simulink subsystem "airframe_aerodynamics"  (R2023b)
settings: Solver=VariableStepAuto  StartTime=0.0  StopTime=10.0  RelTol=1e-3
undefined symbols (not defined in the file): b, c, C_D, C_l, C_L, C_m, C_n, C_Y, p, S
libraries: sharedtransform x1
settings Model: Creator=Victor  LastModifiedBy=Victor

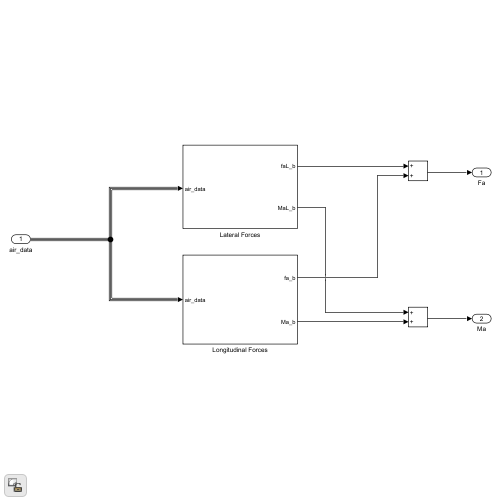
[thumbnail: Simulink's stored preview of the top-level diagram]
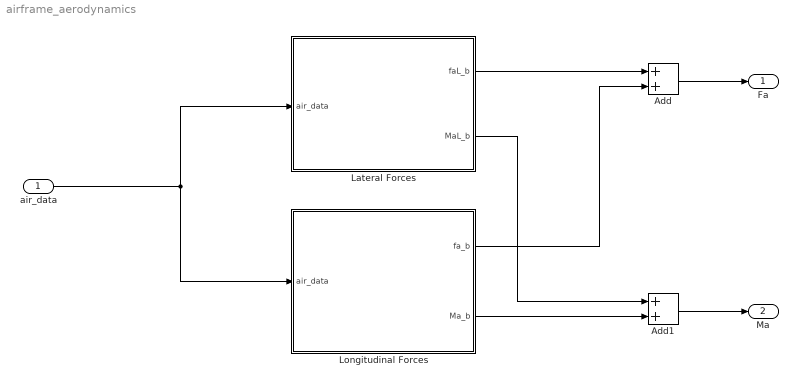
== system airframe_aerodynamics ==
  air_data : Inport
  Add : Sum
  Add1 : Sum
  Lateral Forces : Subsystem
  Longitudinal Forces : Subsystem
  Fa : Outport
  Ma : Outport  Port=2
  wires:
  air_data/1 -> Longitudinal Forces/1(air_data), Lateral Forces/1(air_data)
  Lateral Forces/1(faL_b) -> Add/1
  Longitudinal Forces/1(fa_b) -> Add/2
  Add/1 -> Fa/1
  Lateral Forces/2(MaL_b) -> Add1/1
  Longitudinal Forces/2(Ma_b) -> Add1/2
  Add1/1 -> Ma/1

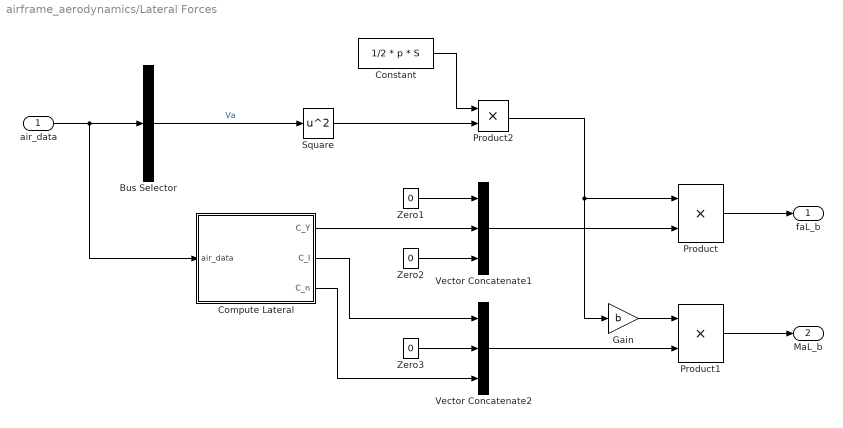
== system airframe_aerodynamics/Lateral Forces ==
  air_data : Inport
  Bus Selector : BusSelector  OutputSignals=target.Va  OutputAsBus=on
  Compute Lateral : Subsystem
  Constant : Constant  Value=1/2 * p * S
  Gain : Gain  Gain=b
  Product : Product
  Product1 : Product
  Product2 : Product
  Square : Math  Operator=square
  Vector Concatenate1 : Concatenate  NumInputs=3
  Vector Concatenate2 : Concatenate  NumInputs=3
  Zero1 : Constant  Value=0  OutDataTypeStr=Inherit: Inherit via back propagation
  Zero2 : Constant  Value=0  OutDataTypeStr=Inherit: Inherit via back propagation
  Zero3 : Constant  Value=0  OutDataTypeStr=Inherit: Inherit via back propagation
  faL_b : Outport
  MaL_b : Outport  Port=2
  wires:
  Bus Selector/1 -> Square/1  "Va"
  Product/1 -> faL_b/1
  air_data/1 -> Compute Lateral/1(air_data), Bus Selector/1
  Zero1/1 -> Vector Concatenate1/1
  Zero2/1 -> Vector Concatenate1/3
  Compute Lateral/1(C_Y) -> Vector Concatenate1/2
  Compute Lateral/3(C_n) -> Vector Concatenate2/3
  Compute Lateral/2(C_l) -> Vector Concatenate2/1
  Zero3/1 -> Vector Concatenate2/2
  Product1/1 -> MaL_b/1
  Square/1 -> Product2/2
  Constant/1 -> Product2/1
  Product2/1 -> Gain/1, Product/1
  Vector Concatenate1/1 -> Product/2
  Vector Concatenate2/1 -> Product1/2
  Gain/1 -> Product1/1

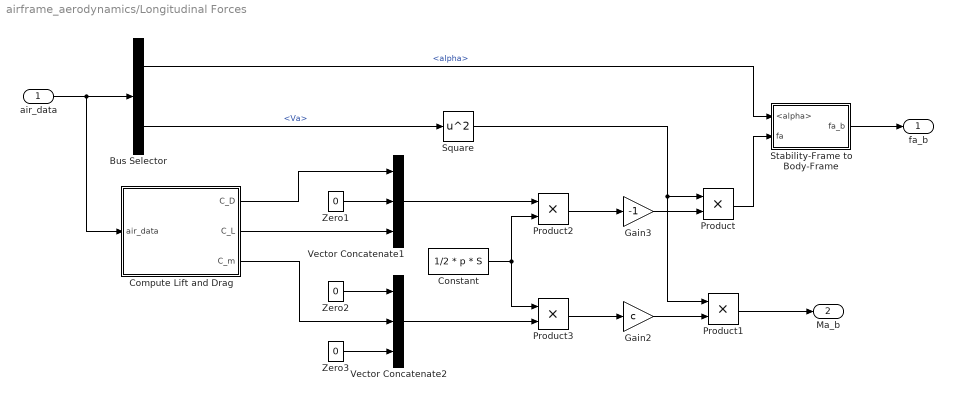
== system airframe_aerodynamics/Longitudinal Forces ==
  air_data : Inport
  Bus Selector : BusSelector  OutputSignals=target.alpha,target.Va
  Compute Lift and Drag : Subsystem
  Constant : Constant  Value=1/2 * p * S
  Gain2 : Gain  Gain=c
  Gain3 : Gain  Gain=-1
  Product{,1..3} (4 alike) : Product
  Square : Math  Operator=square
  Stability-Frame to Body-Frame : Subsystem
  Vector Concatenate1 : Concatenate  NumInputs=3
  Vector Concatenate2 : Concatenate  NumInputs=3
  Zero1 : Constant  Value=0  OutDataTypeStr=Inherit: Inherit via back propagation
  Zero2 : Constant  Value=0  OutDataTypeStr=Inherit: Inherit via back propagation
  Zero3 : Constant  Value=0  OutDataTypeStr=Inherit: Inherit via back propagation
  fa_b : Outport
  Ma_b : Outport  Port=2
  wires:
  air_data/1 -> Bus Selector/1, Compute Lift and Drag/1(air_data)
  Vector Concatenate1/1 -> Product2/1
  Zero1/1 -> Vector Concatenate1/2
  Compute Lift and Drag/1(C_D) -> Vector Concatenate1/1
  Compute Lift and Drag/2(C_L) -> Vector Concatenate1/3
  Vector Concatenate2/1 -> Product3/2
  Zero3/1 -> Vector Concatenate2/3
  Compute Lift and Drag/3(C_m) -> Vector Concatenate2/2
  Product1/1 -> Ma_b/1
  Bus Selector/2 -> Square/1  "<Va>"
  Bus Selector/1 -> Stability-Frame to Body-Frame/1(<alpha>)  "<alpha>"
  Stability-Frame to Body-Frame/1(fa_b) -> fa_b/1
  Zero2/1 -> Vector Concatenate2/1
  Constant/1 -> Product2/2, Product3/1
  Product2/1 -> Gain3/1
  Product3/1 -> Gain2/1
  Gain2/1 -> Product1/2
  Gain3/1 -> Product/2
  Square/1 -> Product1/1, Product/1
  Product/1 -> Stability-Frame to Body-Frame/2(fa)

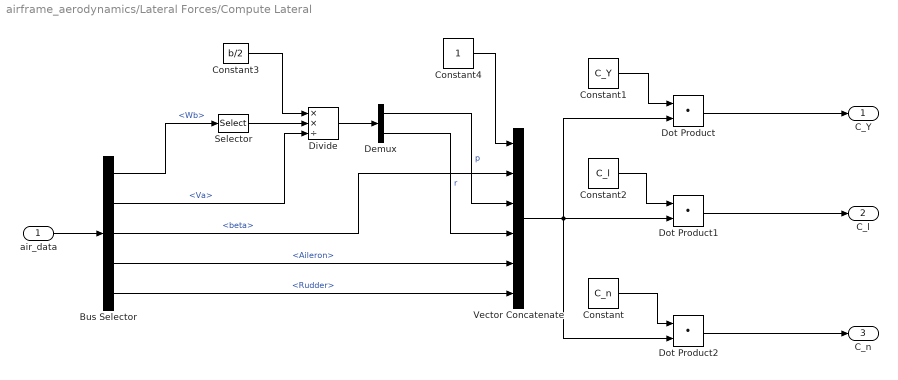
== system airframe_aerodynamics/Lateral Forces/Compute Lateral ==
  air_data : Inport
  Bus Selector : BusSelector  OutputSignals=state.Wb,target.Va,target.beta,control.Aileron,control.Rudder
  Constant : Constant  Value=C_n
  Constant1 : Constant  Value=C_Y
  Constant2 : Constant  Value=C_l
  Constant3 : Constant  Value=b/2
  Constant4 : Constant
  Demux : Demux  Outputs=2
  Divide : Product  Inputs=**/
  Dot Product : DotProduct  OutDataTypeStr=Inherit: Inherit via internal rule
  Dot Product1 : DotProduct  OutDataTypeStr=Inherit: Inherit via internal rule
  Dot Product2 : DotProduct  OutDataTypeStr=Inherit: Inherit via internal rule
  Selector : Selector  InputPortWidth=3  IndexOptions=Index vector (dialog)  Indices=[1 3]  OutputSizes=1
  Vector Concatenate : Concatenate  NumInputs=6
  C_Y : Outport
  C_l : Outport  Port=2
  C_n : Outport  Port=3
  wires:
  air_data/1 -> Bus Selector/1
  Constant1/1 -> Dot Product/1
  Vector Concatenate/1 -> Dot Product2/2, Dot Product1/2, Dot Product/2
  Constant2/1 -> Dot Product1/1
  Dot Product/1 -> C_Y/1
  Dot Product1/1 -> C_l/1
  Dot Product2/1 -> C_n/1
  Selector/1 -> Divide/2
  Constant4/1 -> Vector Concatenate/1
  Demux/1 -> Vector Concatenate/3  "p"
  Demux/2 -> Vector Concatenate/4  "r"
  Divide/1 -> Demux/1
  Constant/1 -> Dot Product2/1
  Bus Selector/1 -> Selector/1  "<Wb>"
  Bus Selector/2 -> Divide/3  "<Va>"
  Bus Selector/3 -> Vector Concatenate/2  "<beta>"
  Bus Selector/4 -> Vector Concatenate/5  "<Aileron>"
  Bus Selector/5 -> Vector Concatenate/6  "<Rudder>"
  Constant3/1 -> Divide/1

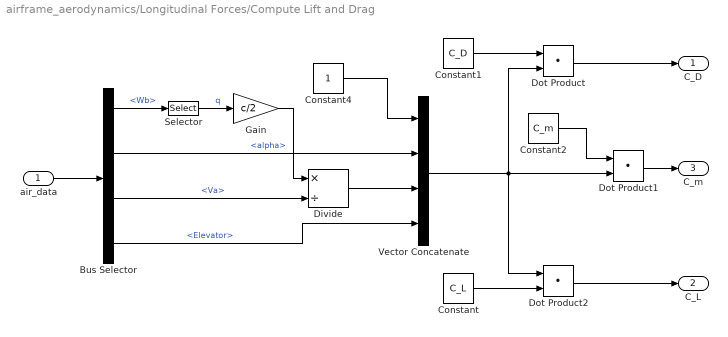
== system airframe_aerodynamics/Longitudinal Forces/Compute Lift and Drag ==
  air_data : Inport
  Bus Selector : BusSelector  OutputSignals=state.Wb,target.alpha,target.Va,control.Elevator
  Constant : Constant  Value=C_L
  Constant1 : Constant  Value=C_D
  Constant2 : Constant  Value=C_m
  Constant4 : Constant
  Divide : Product  Inputs=*/
  Dot Product : DotProduct  OutDataTypeStr=Inherit: Inherit via internal rule
  Dot Product1 : DotProduct  OutDataTypeStr=Inherit: Inherit via internal rule
  Dot Product2 : DotProduct  OutDataTypeStr=Inherit: Inherit via internal rule
  Gain : Gain  Gain=c/2
  Selector : Selector  InputPortWidth=3  IndexOptions=Index vector (dialog)  Indices=[2]  OutputSizes=1
  Vector Concatenate : Concatenate  NumInputs=4
  C_D : Outport
  C_L : Outport  Port=2
  C_m : Outport  Port=3
  wires:
  Constant4/1 -> Vector Concatenate/1
  air_data/1 -> Bus Selector/1
  Bus Selector/2 -> Vector Concatenate/2  "<alpha>"
  Bus Selector/3 -> Divide/2  "<Va>"
  Gain/1 -> Divide/1
  Divide/1 -> Vector Concatenate/3
  Bus Selector/4 -> Vector Concatenate/4  "<Elevator>"
  Constant1/1 -> Dot Product/1
  Vector Concatenate/1 -> Dot Product2/1, Dot Product1/2, Dot Product/2
  Constant/1 -> Dot Product2/2
  Constant2/1 -> Dot Product1/1
  Dot Product/1 -> C_D/1
  Dot Product1/1 -> C_m/1
  Dot Product2/1 -> C_L/1
  Selector/1 -> Gain/1  "q"
  Bus Selector/1 -> Selector/1  "<Wb>"

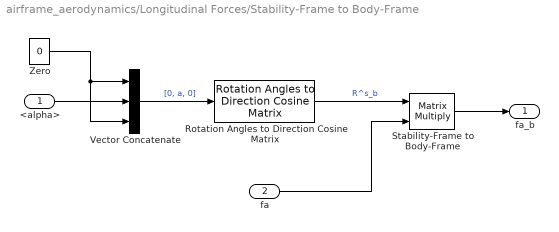
== system airframe_aerodynamics/Longitudinal Forces/Stability-Frame to Body-Frame ==
  <alpha> : Inport
  fa : Inport  Port=2
  Rotation Angles to Direction Cosine Matrix : sharedtransform/Rotation Angles to Direction Cosine Matrix  rotationOrder=ZYX  aMode=aMode
  Stability-Frame to Body-Frame : Product  Multiplication=Matrix(*)
  Vector Concatenate : Concatenate  NumInputs=3
  Zero : Constant  Value=0  OutDataTypeStr=Inherit: Inherit via back propagation
  fa_b : Outport
  wires:
  <alpha>/1 -> Vector Concatenate/2
  Rotation Angles to Direction Cosine Matrix/1 -> Stability-Frame to Body-Frame/1  "R^s_b"
  Zero/1 -> Vector Concatenate/3, Vector Concatenate/1
  Vector Concatenate/1 -> Rotation Angles to Direction Cosine Matrix/1  "[0, a, 0]"
  fa/1 -> Stability-Frame to Body-Frame/2
  Stability-Frame to Body-Frame/1 -> fa_b/1
